simulink model "Fault_Analysis_and_Protection"  (R2025a)
settings: Solver=ode23tb  StartTime=0.0  StopTime=1  RelTol=1e-3
undefined symbols (not defined in the file): D1, Delta
libraries: spsThreePhaseSourceLib x1, spsThreePhaseParallelRLCLoadLib x1, spsThreePhaseVIMeasurementLib x1, spsThreePhaseBreakerLib x1, spsThreePhaseFaultLib x1, spsThreePhaseTransformerTwoWindingsLib x1, sps_lib x1
settings Model: Creator=fahad  LastModifiedBy=fahad

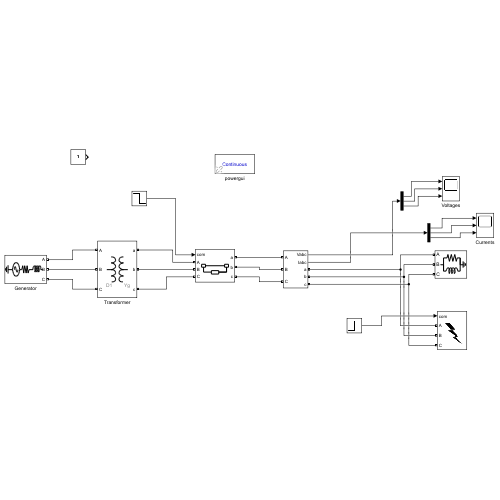
[thumbnail: Simulink's stored preview of the top-level diagram]
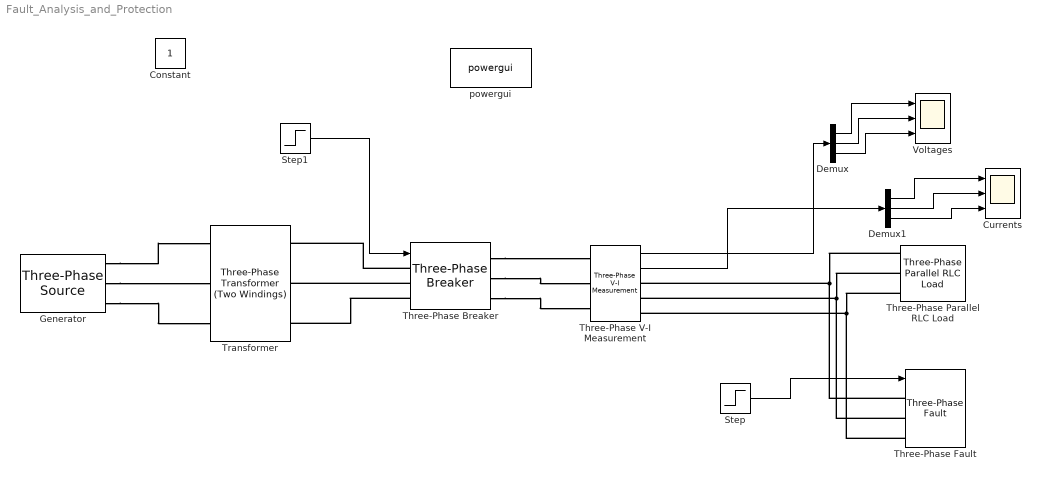
== system Fault_Analysis_and_Protection ==
  Constant : Constant
  Currents : Scope  NumInputPorts=3
      settings: ActiveDisplayYMinimum=-25324.493310683  ActiveDisplayYMaximum=26167.71574957636
  Demux : Demux  Outputs=3
  Demux1 : Demux  Outputs=3
  Generator : spsThreePhaseSourceLib/Three-Phase Source  InternalConnection=Yg  VoltagePhases=off  Voltage=11e3  PhaseAngle=0  Voltage_phases=[25e3 25e3 25e3]/sqrt(3)  PhaseAngles_phases=[0 -120 +120]  Frequency=50  NonIdealSource=on  SpecifyImpedance=on  Resistance=0.8929  Inductance=16.58e-3  ShortCircuitLevel=20e6  BaseVoltage=11e3  XRratio=7  BusType=swing  Pref=10e3  Qref=0  Prefabc=[10e3, 10e3, 10e3]  Qrefabc=[0, 0, 0]  Qmin=-inf  Qmax=inf
  Step : Step  Time=0.1  SampleTime=0
  Step1 : Step  Time=0.15  Before=1  After=0  SampleTime=0
  Three-Phase Parallel RLC Load : spsThreePhaseParallelRLCLoadLib/Three-Phase Parallel RLC Load  LConnTagsString=A|B|C  Configuration=Y (grounded)  NominalVoltage=0.4e3  Vabc=[1e3 1e3 1e3]  Vabcp=[1e3 1e3 1e3]  NominalFrequency=50  UnbalancedPower=off  ActivePower=5e6  InductivePower=20e3  CapacitivePower=0  Pabc=[10e3 9e3 11e3]  QLabc=[100 90 110]  QCabc=[100 90 110]  Pabcp=[10e3 9e3 11e3]  QLabcp=[100 90 110]  QCabcp=[100 90 110]  Measurements=None  LoadType=constant Z
  Three-Phase V-I Measurement : spsThreePhaseVIMeasurementLib/Three-Phase V-I Measurement  VoltageMeasurement=phase-to-ground  SetLabelV=off  LabelV=Vabc  Vpu=off  VpuLL=off  CurrentMeasurement=yes  SetLabelI=off  LabelI=Iabc  Ipu=off  Pbase=100e6  Vbase=500e3  OutputType=Complex  PhasorSimulation=off  PSBequivalent=0
  Three-Phase Breaker : spsThreePhaseBreakerLib/Three-Phase Breaker  InitialState=closed  SwitchA=on  SwitchB=on  SwitchC=on  SwitchTimes="[1/60  5/60]"  External=on  BreakerResistance=0.01  SnubberResistance=1e6  SnubberCapacitance=inf  Measurements=None
  Three-Phase Fault : spsThreePhaseFaultLib/Three-Phase Fault  InitialStates=0  FaultA=on  FaultB=on  FaultC=on  GroundFault=on  SwitchTimes="[1/60  5/60]"  External=on  SwitchStatus=NaN  FaultResistance=0.001  GroundResistance=0.01  SnubberResistance=1e6  SnubberCapacitance=inf  Measurements=None
  Transformer : spsThreePhaseTransformerTwoWindingsLib/Three-Phase Transformer (Two Windings)  Winding1Connection=Delta (D1)  Winding2Connection=Yg  CoreType=Three single-phase transformers  SetSaturation=off  Hysteresis=off  DataFile='hysteresis'  SetInitialFlux=off  Measurements=None  UNITS=pu  NominalPower=[ 10e6 , 50 ]  Winding1=[ 11e3 , 0.002 , 0.08 ]  Winding2=[ 0.4e3 , 0.002 , 0.08 ]  Rm=500  Lm=500  L0=0.5  Saturation=[ 0,0 ; 0.0024,1.2 ; 1.0,1.52 ]  InitialFluxes=[ 0.8 , -0.8 , 0.7 ]  BreakLoop=off  DiscreteSolver=Trapezoidal iterative  DataType=off  TransfoNumber=1
  Voltages : Scope  NumInputPorts=3
      settings: ActiveDisplayYMinimum=-292.48737856940261  ActiveDisplayYMaximum=293.01658266460146
  powergui : sps_lib/powergui  Priority=1  SimulationMode=Continuous  SampleTime=50e-6  frequency=60  Iterations=50  frequencyindice=50  Pbase=100e6  ErrMax=1e-4  UnitsV=kV  UnitsW=MW  buscounter=0  FunctionMessages=off  echomessages=off  EnableUseOfTLC=off  CurrentSourceSwitches=off  DisableSnubberDevices=off  DisableRonSwitches=off  DisableVfSwitches=off  DisplayEquations=off  AutomaticDiscreteSolvers=off  SolverType=Tustin/Backward Euler (TBE)  Interpol=off  ExternalGateDelay=off  methode=off  Ts=100  x0status=blocks  SPID=on  SwTol=0  HookPort=off  NonlinearTolerance=1e-4  nMaxIteration=100  ContinueOnMaxIteration=off  RestoreLinks=warning  ResistiveCurrentMeasurement=off  Frange=[0:2:500]  Ylog=off  Xlog=on  ShowGrid=off  save=off  variable=ZData  structure=0  ZoomFFT=off  StartTime=0.0  cycles=1  DisplayStyle=1  fundamental=60  FreqAxis=off  MaxFrequency=1000  frequencyindicesteady=1  RmsSteady=1  display=off
  wires:
  Three-Phase V-I Measurement/1 -> Demux/1
  Demux/1 -> Voltages/1
  Demux/2 -> Voltages/2
  Demux/3 -> Voltages/3
  Three-Phase V-I Measurement/2 -> Demux1/1
  Demux1/1 -> Currents/1
  Demux1/2 -> Currents/2
  Demux1/3 -> Currents/3
  Step/1 -> Three-Phase Fault/1
  Step1/1 -> Three-Phase Breaker/1
  connections:
  Generator/RConn1 -- Transformer/LConn1
  Generator/RConn2 -- Transformer/LConn2
  Generator/RConn3 -- Transformer/LConn3
  Three-Phase Parallel RLC Load/LConn1 -- Three-Phase Fault/LConn1 -- Three-Phase V-I Measurement/RConn1
  Three-Phase Parallel RLC Load/LConn2 -- Three-Phase Fault/LConn2 -- Three-Phase V-I Measurement/RConn2
  Three-Phase Parallel RLC Load/LConn3 -- Three-Phase Fault/LConn3 -- Three-Phase V-I Measurement/RConn3
  Three-Phase Breaker/LConn1 -- Transformer/RConn1
  Three-Phase Breaker/LConn2 -- Transformer/RConn2
  Three-Phase Breaker/LConn3 -- Transformer/RConn3
  Three-Phase Breaker/RConn1 -- Three-Phase V-I Measurement/LConn1
  Three-Phase Breaker/RConn2 -- Three-Phase V-I Measurement/LConn2
  Three-Phase Breaker/RConn3 -- Three-Phase V-I Measurement/LConn3
